simulink model "Multidifusor1"  (R2023a)
settings: Solver=VariableStepAuto  StartTime=0.0  StopTime=10.0  RelTol=1e-3
undefined symbols (not defined in the file): m, n
settings Model: Creator=santi  LastModifiedBy=santi

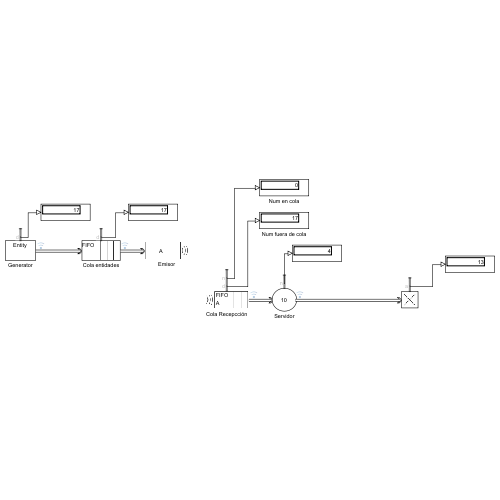
[thumbnail: Simulink's stored preview of the top-level diagram]
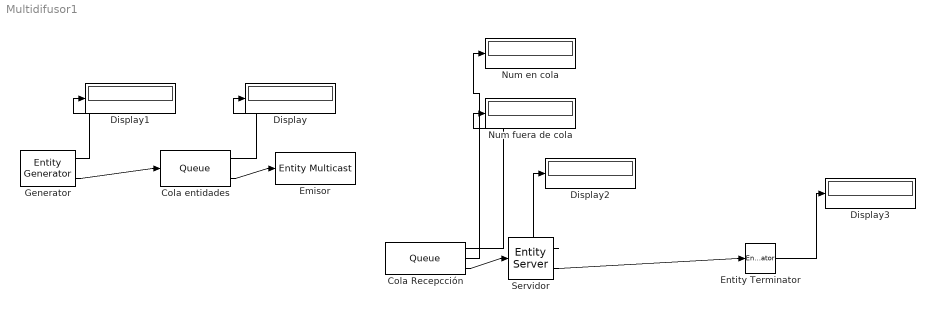
== system Multidifusor1 ==
  Cola Recepcción : Queue  OutputPortMessageModes=n,n,m  EntityArrivalSource=Multicast  NumberEntitiesDeparted=on  NumberEntitiesInBlock=on
      settings: OutputPortMap=o0,o1,o5
  Cola entidades : Queue  InputPortMessageModes=m  OutputPortMessageModes=n,m  NumberEntitiesDeparted=on
      settings: OutputPortMap=o0,o5
  Display{,1..3} (4 alike) : Display
  Emisor : EntityMulticast  Tag=A  InputPortMessageModes=m
  Entity Terminator : EntityTerminator  InputPortMessageModes=m  NumberEntitiesArrived=on
      settings: OutputPortMap=o0
  Generator : EntityGenerator  OutputPortMessageModes=n,m  TimeSource=MATLAB action  NumberEntitiesDeparted=on  EntityType=Structured  EntityTypeName=Entity
      settings: OutputPortMap=o0,o3
  Num en cola : Display
  Num fuera de cola : Display
  Servidor : EntityServer  InputPortMessageModes=m  OutputPortMessageModes=n,m  Capacity=10  ServiceTimeValue=2  NumberEntitiesInBlock=on
      settings: OutputPortMap=o1,o9
  wires:
  Generator/2 -> Cola entidades/1
  Cola entidades/2 -> Emisor/1
  Cola Recepcción/3 -> Servidor/1
  Servidor/2 -> Entity Terminator/1
  Generator/1 -> Display1/1
  Cola entidades/1 -> Display/1
  Cola Recepcción/1 -> Num fuera de cola/1
  Entity Terminator/1 -> Display3/1
  Cola Recepcción/2 -> Num en cola/1
  Servidor/1 -> Display2/1
